simulink model "CylindricalCellModel"  (R2020b)
settings: Solver=VariableStepAuto  StartTime=0.0  StopTime=Model.Time(end)  RelTol=1e-3
libraries: fl_lib x12, nesl_utility x3
settings Model: Creator=Max  LastModifiedBy=Max
settings DataIOCC: ExternalInput=Model.Ohmic  LoadExternalInput=on

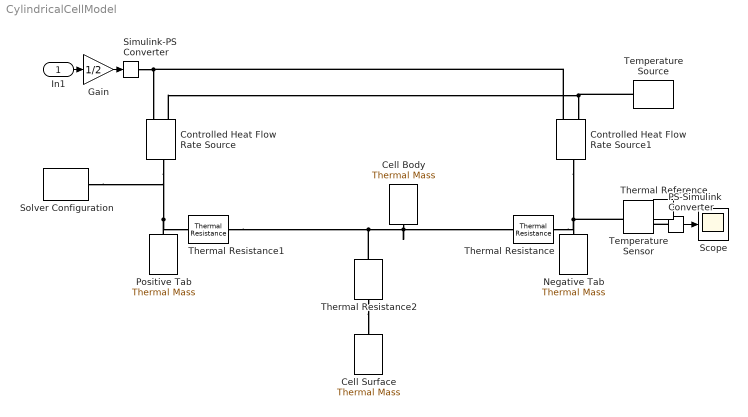
== system CylindricalCellModel ==
  In1 : Inport
  Cell Body : fl_lib/Thermal/Thermal Elements/Thermal Mass  mass=Cell.Mass kg  sp_heat=Cell.Cp J/kg/K  T_specify=off  T_priority=High  T=300 K  T_nominal_specify=off  T_nominal_unit=K  T_nominal_value=1  Q_specify=off  Q_priority=None  Q=0 W  Q_nominal_specify=off  Q_nominal_unit=W  Q_nominal_value=1
  Cell Surface : fl_lib/Thermal/Thermal Elements/Thermal Mass  mass=4 g  sp_heat=Cell.Cp J/kg/K  T_specify=off  T_priority=High  T=300 K  T_nominal_specify=off  T_nominal_unit=K  T_nominal_value=1  Q_specify=off  Q_priority=None  Q=0 W  Q_nominal_specify=off  Q_nominal_unit=W  Q_nominal_value=1
  Controlled Heat Flow Rate Source : fl_lib/Thermal/Thermal Sources/Controlled Heat Flow Rate Source
  Controlled Heat Flow Rate Source1 : fl_lib/Thermal/Thermal Sources/Controlled Heat Flow Rate Source
  Gain : Gain  Gain=1/2
  Negative Tab : fl_lib/Thermal/Thermal Elements/Thermal Mass  mass=2 g  sp_heat=Cell.Cp J/kg/K  T_specify=off  T_priority=High  T=300 K  T_nominal_specify=off  T_nominal_unit=K  T_nominal_value=1  Q_specify=off  Q_priority=None  Q=0 W  Q_nominal_specify=off  Q_nominal_unit=W  Q_nominal_value=1
  PS-Simulink Converter : nesl_utility/PS-Simulink Converter  PhysicalDomain=network_engine_domain  SubClassName=ps_output  LeftPortType=input  RightPortType=output  PseudoPeriodic=off  Frequencies=[]  Unit=inherit  AffineConversion=off
  Positive Tab : fl_lib/Thermal/Thermal Elements/Thermal Mass  mass=2 g  sp_heat=Cell.Cp J/kg/K  T_specify=off  T_priority=High  T=300 K  T_nominal_specify=off  T_nominal_unit=K  T_nominal_value=1  Q_specify=off  Q_priority=None  Q=0 W  Q_nominal_specify=off  Q_nominal_unit=W  Q_nominal_value=1
  Scope : Scope
  Simulink-PS Converter : nesl_utility/Simulink-PS Converter  PhysicalDomain=network_engine_domain  SubClassName=ps_input  LeftPortType=input  RightPortType=output  PseudoPeriodic=off  Frequencies=[]  NoiseDistribution=none  NoiseParameters=[]  Unit=1  AffineConversion=off  FilteringAndDerivatives=provide  SimscapeFilterOrder=1  InputFilterTimeConstant=0.001  UdotUserProvided=0
  Solver Configuration : nesl_utility/Solver Configuration  PhysicalDomain=network_engine_domain  SubClassName=solver  LeftPortType=input  RightPortType=generic  Tones=[]  Harmonics=[]  SimulateNoise=off  Profile=off  UseLocalSampling=off  EnableSwitchedLinearOptims=on  FrequencyDomain=off  UseCCode=off  RelTol=0.001  AbsTol=1e-06  MinStep=1e-09  ToWorkspace=off  RevertToSquareIcSolve=off  NumHomotopyIterations=100  PhasorMode=off  PhasorModeNumHarmonics=1  DoDC=off  ResidualTolerance=1e-09  UseLocalSolver=off  LocalSolverChoice=NE_BACKWARD_EULER_ADVANCER  LocalSolverSampleTime=0.001  DoFixedCost=off  MaxNonlinIter=3  MaxModeIter=2  ComputeImpulses=off  ImpulseIterations=2  LinearAlgebra=auto  EquationFormulation=NE_TIME_EF  DelaysMemoryBudget=1024  AutomaticFiltering=on  FilteringTimeConstant=0.001  PartitionStorageMethod=AS_NEEDED  PartitionMemoryBudget=1024  PartitionMethod=ROBUST
  Temperature Sensor : fl_lib/Thermal/Thermal Sensors/Temperature Sensor
  Temperature Source : fl_lib/Thermal/Thermal Sources/Temperature Source  temperature=35 degC
  Thermal Reference : fl_lib/Thermal/Thermal Elements/Thermal Reference
  Thermal Resistance : fl_lib/Thermal/Thermal Elements/Thermal Resistance  resistance=Cell.R_Axial K/W  T_specify=off  T_priority=None  T=0 K  T_nominal_specify=off  T_nominal_unit=K  T_nominal_value=1  Q_specify=off  Q_priority=None  Q=0 W  Q_nominal_specify=off  Q_nominal_unit=W  Q_nominal_value=1
      settings: SourceProductBaseCode=SS
  Thermal Resistance1 : fl_lib/Thermal/Thermal Elements/Thermal Resistance  resistance=Cell.R_Axial K/W  T_specify=off  T_priority=None  T=0 K  T_nominal_specify=off  T_nominal_unit=K  T_nominal_value=1  Q_specify=off  Q_priority=None  Q=0 W  Q_nominal_specify=off  Q_nominal_unit=W  Q_nominal_value=1
      settings: SourceProductBaseCode=SS
  Thermal Resistance2 : fl_lib/Thermal/Thermal Elements/Thermal Resistance  resistance=Cell.R_Radial K/W  T_specify=off  T_priority=None  T=0 K  T_nominal_specify=off  T_nominal_unit=K  T_nominal_value=1  Q_specify=off  Q_priority=None  Q=0 W  Q_nominal_specify=off  Q_nominal_unit=W  Q_nominal_value=1
      settings: SourceProductBaseCode=SS
  wires:
  In1/1 -> Gain/1
  Gain/1 -> Simulink-PS Converter/1
  PS-Simulink Converter/1 -> Scope/1
  connections:
  Thermal Resistance/RConn1 -- Temperature Sensor/LConn1 -- Controlled Heat Flow Rate Source1/LConn1 -- Negative Tab/LConn1
  Positive Tab/LConn1 -- Solver Configuration/RConn1 -- Controlled Heat Flow Rate Source/LConn1 -- Thermal Resistance1/RConn1
  Thermal Resistance2/RConn1 -- Cell Surface/LConn1
  Thermal Resistance1/LConn1 -- Cell Body/LConn1 -- Thermal Resistance/LConn1 -- Thermal Resistance2/LConn1
  Simulink-PS Converter/RConn1 -- Controlled Heat Flow Rate Source1/RConn1 -- Controlled Heat Flow Rate Source/RConn1
  Controlled Heat Flow Rate Source/RConn2 -- Temperature Source/LConn1 -- Controlled Heat Flow Rate Source1/RConn2
  Thermal Reference/LConn1 -- Temperature Sensor/RConn1
  PS-Simulink Converter/LConn1 -- Temperature Sensor/RConn2
